simulink model "s_6dof2016a"  (R2016a)
settings: Solver=VariableStepAuto  SolverMode=SingleTasking  StartTime=0.0  StopTime=90  RelTol=1e-3
(part 2 of 2)

== system s_6dof2016a/Subsystem1/B/b513 ==
  t5 : Inport
  t2 : Inport  Port=2
  t3 : Inport  Port=3
  t4 : Inport  Port=4
  Constant4 : Constant  Value=-1
  Product : Product
  b1 : Subsystem
  b513 : Outport
  wires:
  t5/1 -> b1/3(t5)
  Constant4/1 -> Product/2
  b1/1(b315) -> Product/1
  t4/1 -> b1/2(t4)
  Product/1 -> b513/1
  t2/1 -> b1/1(t2)
  t3/1 -> b1/4(t3)

== system s_6dof2016a/Subsystem1/B/b514 ==
  t2 : Inport
  t3 : Inport  Port=2
  t4 : Inport  Port=3
  Constant3 : Constant  Value=-1
  Product : Product
  b1 : Subsystem
  b514 : Outport
  wires:
  Constant3/1 -> Product/2
  t4/1 -> b1/3(t4)
  t2/1 -> b1/1(t2)
  b1/1(b415) -> Product/1
  Product/1 -> b514/1
  t3/1 -> b1/2(t3)

== system s_6dof2016a/Subsystem1/B/b523 ==
  t5 : Inport
  Constant3 : Constant  Value=-1
  Product1 : Product
  b1 : Subsystem
  b523 : Outport
  wires:
  b1/1(b325) -> Product1/1
  t5/1 -> b1/1(t5)
  Constant3/1 -> Product1/2
  Product1/1 -> b523/1

== system s_6dof2016a/Subsystem1/B/b524 ==
  t4 : Inport
  Constant3 : Constant  Value=-1
  Product1 : Product
  b1 : Subsystem
  b524 : Outport
  wires:
  b1/1(b425) -> Product1/1
  t4/1 -> b1/1(t4)
  Product1/1 -> b524/1
  Constant3/1 -> Product1/2

== system s_6dof2016a/Subsystem1/B/b534 ==
  t4 : Inport
  Constant3 : Constant  Value=-1
  Product1 : Product
  b1 : Subsystem
  b524 : Outport
  wires:
  Constant3/1 -> Product1/2
  Product1/1 -> b524/1
  t4/1 -> b1/1(t4)
  b1/1(b425) -> Product1/1

== system s_6dof2016a/Subsystem1/C/c12 ==
  t2 : Inport
  t3 : Inport  Port=2
  Add1 : Sum  Inputs=+++
  Add2 : Sum
  Product1 : Product
  Product3 : Product
  Product4 : Product
  Trigonometric Function1 : Trigonometry  Operator=cos
  Trigonometric Function4 : Trigonometry
  Trigonometric Function5 : Trigonometry
  c2 : Constant  Value=0.69
  c3 : Constant  Value=0.134
  c4 : Constant  Value=-0.0238
  c12 : Outport
  wires:
  Product1/1 -> Add1/1
  Product4/1 -> Add1/3
  Trigonometric Function1/1 -> Product1/2
  Trigonometric Function4/1 -> Product3/2
  Product3/1 -> Add1/2
  t2/1 -> Trigonometric Function5/1, Add2/1, Trigonometric Function1/1
  Add2/1 -> Trigonometric Function4/1
  Trigonometric Function5/1 -> Product4/2
  t3/1 -> Add2/2
  c2/1 -> Product1/1
  c3/1 -> Product3/1
  c4/1 -> Product4/1
  Add1/1 -> c12/1

== system s_6dof2016a/Subsystem1/C/c13 ==
  t2 : Inport
  "t3 " : Inport  Port=2
  Product1 : Product
  Product2 : Product
  Sum2 : Sum  Inputs=|++
  Sum3 : Sum  Inputs=|++
  Trigonometric Function : Trigonometry
  Trigonometric Function1 : Trigonometry  Operator=cos
  b1 : Constant  Value=0.267
  b2 : Constant  Value=-0.00758
  b123 : Outport
  wires:
  Trigonometric Function/1 -> Product2/2
  Product1/1 -> Sum3/2
  Sum3/1 -> b123/1
  Trigonometric Function1/1 -> Product1/2
  Sum2/1 -> Trigonometric Function1/1, Trigonometric Function/1
  b1/1 -> Product2/1
  Product2/1 -> Sum3/1
  b2/1 -> Product1/1
  "t3 "/1 -> Sum2/2
  t2/1 -> Sum2/1

== system s_6dof2016a/Subsystem1/C/c21 ==
  t2 : Inport
  t3 : Inport  Port=2
  Product1 : Product
  b112 : Subsystem
  c2 : Constant  Value=-0.5
  c21 : Outport
  wires:
  c2/1 -> Product1/2
  Product1/1 -> c21/1
  b112/1(b112) -> Product1/1
  t3/1 -> b112/2(t3)
  t2/1 -> b112/1(t2)

== system s_6dof2016a/Subsystem1/C/c23 ==
  t3 : Inport
  Product2 : Product
  b223 : Subsystem
  c2 : Constant  Value=0.5
  c23 : Outport
  wires:
  b223/1(b223) -> Product2/1
  t3/1 -> b223/1(t3)
  c2/1 -> Product2/2
  Product2/1 -> c23/1

== system s_6dof2016a/Subsystem1/C/c31 ==
  t2 : Inport
  t3 : Inport  Port=2
  Product2 : Product
  b113 : Subsystem
  c2 : Constant  Value=-0.5
  c31 : Outport
  wires:
  b113/1(b113) -> Product2/1
  t2/1 -> b113/1(t2)
  c2/1 -> Product2/2
  Product2/1 -> c31/1
  t3/1 -> b113/2(t3)

== system s_6dof2016a/Subsystem1/C/c32 ==
  t3 : Inport
  Product2 : Product
  c2 : Subsystem
  c3 : Constant  Value=-1
  c32 : Outport
  wires:
  c3/1 -> Product2/2
  c2/1(c23) -> Product2/1
  t3/1 -> c2/1(t3)
  Product2/1 -> c32/1

== system s_6dof2016a/Subsystem1/C/c34 ==
  t4 : Inport
  t5 : Inport  Port=2
  Product2 : Product  Inputs=3
  Trigonometric Function1 : Trigonometry  Operator=cos
  Trigonometric Function4 : Trigonometry
  c2 : Constant  Value=-0.00125
  c34 : Outport
  wires:
  Product2/1 -> c34/1
  Trigonometric Function1/1 -> Product2/2
  c2/1 -> Product2/1
  Trigonometric Function4/1 -> Product2/3
  t4/1 -> Trigonometric Function1/1
  t5/1 -> Trigonometric Function4/1

== system s_6dof2016a/Subsystem1/C/c35 ==
  t4 : Inport
  t5 : Inport  Port=2
  Product2 : Product  Inputs=3
  Trigonometric Function1 : Trigonometry  Operator=cos
  Trigonometric Function4 : Trigonometry
  c2 : Constant  Value=-0.00125
  c34 : Outport
  wires:
  Product2/1 -> c34/1
  Trigonometric Function1/1 -> Product2/2
  c2/1 -> Product2/1
  Trigonometric Function4/1 -> Product2/3
  t4/1 -> Trigonometric Function1/1
  t5/1 -> Trigonometric Function4/1

== system s_6dof2016a/Subsystem1/C/c41 ==
  t2 : Inport
  t3 : Inport  Port=2
  t4 : Inport  Port=3
  t5 : Inport  Port=4
  Product2 : Product
  b114 : Subsystem
  c2 : Constant  Value=-0.5
  c41 : Outport
  wires:
  c2/1 -> Product2/2
  t2/1 -> b114/3(t2)
  b114/1(b114) -> Product2/1
  t4/1 -> b114/1(t4)
  Product2/1 -> c41/1
  t3/1 -> b114/4(t3)
  t5/1 -> b114/2(t5)

== system s_6dof2016a/Subsystem1/C/c42 ==
  t3 : Inport
  t4 : Inport  Port=2
  t5 : Inport  Port=3
  Product2 : Product
  b224 : Subsystem
  c2 : Constant  Value=-0.5
  c42 : Outport
  wires:
  t3/1 -> b224/3(t3)
  c2/1 -> Product2/2
  b224/1(b224) -> Product2/1
  t4/1 -> b224/1(t4)
  t5/1 -> b224/2(t5)
  Product2/1 -> c42/1

== system s_6dof2016a/Subsystem1/C/c51 ==
  t2 : Inport
  t3 : Inport  Port=2
  t4 : Inport  Port=3
  t5 : Inport  Port=4
  Product2 : Product
  b115 : Subsystem
  c2 : Constant  Value=-0.5
  c51 : Outport
  wires:
  t5/1 -> b115/2(t5)
  c2/1 -> Product2/2
  b115/1(b115) -> Product2/1
  Product2/1 -> c51/1
  t3/1 -> b115/4(t3)
  t2/1 -> b115/3(t2)
  t4/1 -> b115/1(t4)

== system s_6dof2016a/Subsystem1/C/c52 ==
  t3 : Inport
  t4 : Inport  Port=2
  t5 : Inport  Port=3
  Product2 : Product
  b225 : Subsystem
  c2 : Constant  Value=-0.5
  c52 : Outport
  wires:
  t4/1 -> b225/1(t4)
  b225/1(b225) -> Product2/1
  c2/1 -> Product2/2
  t3/1 -> b225/3(t3)
  Product2/1 -> c52/1
  t5/1 -> b225/2(t5)

== system s_6dof2016a/Subsystem1/C/c53 ==
  t5 : Inport
  Product2 : Product
  b523 : Subsystem
  c2 : Constant  Value=0.5
  c53 : Outport
  wires:
  c2/1 -> Product2/2
  b523/1(b523) -> Product2/1
  t5/1 -> b523/1(t5)
  Product2/1 -> c53/1

== system s_6dof2016a/Subsystem2/Subsystem/a11 ==
  t2 : Inport
  t3 : Inport  Port=2
  Constant3 : Constant  Value=2.57
  Constant4 : Constant  Value=1.38
  Constant5 : Constant  Value=0.3
  Constant6 : Constant  Value=0.744
  Product1 : Product  Inputs=3
  Product2 : Product  Inputs=3
  Product3 : Product  Inputs=3
  Sum : Sum  Inputs=|++
  Sum2 : Sum  Inputs=|++++
  Trigonometric Function1 : Trigonometry  Operator=cos
  Trigonometric Function2 : Trigonometry  Operator=cos
  Trigonometric Function3 : Trigonometry
  Trigonometric Function4 : Trigonometry
  Trigonometric Function5 : Trigonometry
  Trigonometric Function6 : Trigonometry  Operator=cos
  a11 : Outport
  wires:
  Trigonometric Function5/1 -> Product3/1
  Product2/1 -> Sum2/3
  t2/1 -> Trigonometric Function6/1, Sum/1, Trigonometric Function3/1, Trigonometric Function2/1, Trigonometric Function1/1
  t3/1 -> Trigonometric Function4/1, Sum/2
  Constant5/1 -> Product2/3
  Trigonometric Function4/1 -> Product2/2
  Product1/1 -> Sum2/2
  Trigonometric Function3/1 -> Product2/1
  Sum2/1 -> a11/1
  Constant6/1 -> Product3/3
  Trigonometric Function6/1 -> Product3/2
  Sum/1 -> Trigonometric Function5/1
  Constant3/1 -> Sum2/1
  Trigonometric Function1/1 -> Product1/1
  Constant4/1 -> Product1/3
  Trigonometric Function2/1 -> Product1/2
  Product3/1 -> Sum2/4

== system s_6dof2016a/Subsystem2/Subsystem/a12 ==
  t2 : Inport
  t3 : Inport  Port=2
  Constant3 : Constant  Value=0.69
  Constant4 : Constant  Value=0.134
  Constant5 : Constant  Value=0.0238
  Product1 : Product
  Product2 : Product
  Product3 : Product
  Sum1 : Sum  Inputs=|++
  Sum3 : Sum  Inputs=|+-+
  Trigonometric Function1 : Trigonometry
  Trigonometric Function2 : Trigonometry  Operator=cos
  Trigonometric Function3 : Trigonometry  Operator=cos
  a12 : Outport
  wires:
  Constant4/1 -> Product2/1
  t2/1 -> Trigonometric Function3/1, Sum1/1, Trigonometric Function1/1
  Trigonometric Function1/1 -> Product1/2
  Product2/1 -> Sum3/2
  Constant5/1 -> Product3/1
  Product1/1 -> Sum3/1
  Product3/1 -> Sum3/3
  Constant3/1 -> Product1/1
  Sum3/1 -> a12/1
  Trigonometric Function3/1 -> Product3/2
  Sum1/1 -> Trigonometric Function2/1
  Trigonometric Function2/1 -> Product2/2
  t3/1 -> Sum1/2

== system s_6dof2016a/Subsystem2/Subsystem/a13 ==
  "t2 " : Inport
  "t3 " : Inport  Port=2
  Constant3 : Constant  Value=0.134
  Constant4 : Constant  Value=0.00397
  Product : Product
  Product1 : Product
  Sum1 : Sum  Inputs=|++
  Sum3 : Sum  Inputs=|--
  Trigonometric Function1 : Trigonometry  Operator=cos
  Trigonometric Function2 : Trigonometry
  "a13 " : Outport
  wires:
  Product/1 -> Sum3/1
  Sum1/1 -> Trigonometric Function2/1, Trigonometric Function1/1
  Product1/1 -> Sum3/2
  Constant4/1 -> Product1/1
  Constant3/1 -> Product/1
  "t2 "/1 -> Sum1/2
  Trigonometric Function2/1 -> Product1/2
  Trigonometric Function1/1 -> Product/2
  Sum3/1 -> "a13 "/1
  "t3 "/1 -> Sum1/1

== system s_6dof2016a/Subsystem2/Subsystem/a21 ==
  t2 : Inport
  t3 : Inport  Port=2
  Constant3 : Constant  Value=0.69
  Constant4 : Constant  Value=0.134
  Constant5 : Constant  Value=0.0238
  Product1 : Product
  Product2 : Product
  Product3 : Product
  Sum1 : Sum  Inputs=|++
  Sum3 : Sum  Inputs=|+-+
  Trigonometric Function1 : Trigonometry
  Trigonometric Function2 : Trigonometry  Operator=cos
  Trigonometric Function3 : Trigonometry  Operator=cos
  a12 : Outport
  wires:
  Constant4/1 -> Product2/1
  t2/1 -> Trigonometric Function3/1, Sum1/1, Trigonometric Function1/1
  Trigonometric Function1/1 -> Product1/2
  Product2/1 -> Sum3/2
  Constant5/1 -> Product3/1
  Product1/1 -> Sum3/1
  Product3/1 -> Sum3/3
  Constant3/1 -> Product1/1
  Sum3/1 -> a12/1
  Trigonometric Function3/1 -> Product3/2
  Sum1/1 -> Trigonometric Function2/1
  Trigonometric Function2/1 -> Product2/2
  t3/1 -> Sum1/2

== system s_6dof2016a/Subsystem2/Subsystem/a22 ==
  t3 : Inport
  Constant3 : Constant  Value=6.79
  Constant4 : Constant  Value=0.744
  Product1 : Product
  Sum1 : Sum  Inputs=|++
  Trigonometric Function1 : Trigonometry
  a22 : Outport
  wires:
  t3/1 -> Trigonometric Function1/1
  Trigonometric Function1/1 -> Product1/1
  Constant4/1 -> Product1/2
  Product1/1 -> Sum1/1
  Sum1/1 -> a22/1
  Constant3/1 -> Sum1/2

== system s_6dof2016a/Subsystem2/Subsystem/a23 ==
  "t3 " : Inport
  Constant3 : Constant  Value=0.333
  Constant4 : Constant  Value=0.372
  Constant5 : Constant  Value=0.011
  Product1 : Product
  Product2 : Product
  Sum1 : Sum  Inputs=|++-
  Trigonometric Function2 : Trigonometry
  Trigonometric Function3 : Trigonometry  Operator=cos
  a23 : Outport
  wires:
  Constant5/1 -> Product1/1
  Trigonometric Function3/1 -> Product1/2
  Product2/1 -> Sum1/2
  Constant3/1 -> Sum1/1
  "t3 "/1 -> Trigonometric Function3/1, Trigonometric Function2/1
  Product1/1 -> Sum1/3
  Trigonometric Function2/1 -> Product2/2
  Constant4/1 -> Product2/1
  Sum1/1 -> a23/1

== system s_6dof2016a/Subsystem2/Subsystem/a31 ==
  "t2 " : Inport
  "t3 " : Inport  Port=2
  Constant3 : Constant  Value=0.134
  Constant4 : Constant  Value=0.00397
  Product : Product
  Product1 : Product
  Sum1 : Sum  Inputs=|++
  Sum3 : Sum  Inputs=|--
  Trigonometric Function1 : Trigonometry  Operator=cos
  Trigonometric Function2 : Trigonometry
  "a13 " : Outport
  wires:
  Product/1 -> Sum3/1
  Sum1/1 -> Trigonometric Function2/1, Trigonometric Function1/1
  Product1/1 -> Sum3/2
  Constant4/1 -> Product1/1
  Constant3/1 -> Product/1
  "t2 "/1 -> Sum1/2
  Trigonometric Function2/1 -> Product1/2
  Trigonometric Function1/1 -> Product/2
  Sum3/1 -> "a13 "/1
  "t3 "/1 -> Sum1/1

== system s_6dof2016a/Subsystem2/Subsystem/a32 ==
  "t3 " : Inport
  Constant3 : Constant  Value=0.333
  Constant4 : Constant  Value=0.372
  Constant5 : Constant  Value=0.011
  Product1 : Product
  Product2 : Product
  Sum1 : Sum  Inputs=|++-
  Trigonometric Function2 : Trigonometry
  Trigonometric Function3 : Trigonometry  Operator=cos
  a23 : Outport
  wires:
  Constant5/1 -> Product1/1
  Trigonometric Function3/1 -> Product1/2
  Product2/1 -> Sum1/2
  Constant3/1 -> Sum1/1
  "t3 "/1 -> Trigonometric Function3/1, Trigonometric Function2/1
  Product1/1 -> Sum1/3
  Trigonometric Function2/1 -> Product2/2
  Constant4/1 -> Product2/1
  Sum1/1 -> a23/1

== system s_6dof2016a/Subsystem2/Subsystem/a34 ==
  t4 : Inport
  t5 : Inport  Port=2
  Product1 : Product  Inputs=3
  Trigonometric Function1 : Trigonometry
  Trigonometric Function2 : Trigonometry
  a1 : Constant  Value=-0.00125
  a34 : Outport
  wires:
  Trigonometric Function2/1 -> Product1/3
  t4/1 -> Trigonometric Function1/1
  Trigonometric Function1/1 -> Product1/2
  Product1/1 -> a34/1
  a1/1 -> Product1/1
  t5/1 -> Trigonometric Function2/1

== system s_6dof2016a/Subsystem2/Subsystem/a35 ==
  t5 : Inport
  "t4 " : Inport  Port=2
  Product1 : Product  Inputs=3
  Trigonometric Function1 : Trigonometry  Operator=cos
  Trigonometric Function2 : Trigonometry  Operator=cos
  a1 : Constant  Value=0.00125
  a35 : Outport
  wires:
  a1/1 -> Product1/1
  Trigonometric Function1/1 -> Product1/2
  Trigonometric Function2/1 -> Product1/3
  "t4 "/1 -> Trigonometric Function1/1
  Product1/1 -> a35/1
  t5/1 -> Trigonometric Function2/1

== system s_6dof2016a/Subsystem2/Subsystem/a43 ==
  t4 : Inport
  t5 : Inport  Port=2
  Product1 : Product  Inputs=3
  Trigonometric Function1 : Trigonometry
  Trigonometric Function2 : Trigonometry
  a1 : Constant  Value=-0.00125
  a34 : Outport
  wires:
  t5/1 -> Trigonometric Function2/1
  a1/1 -> Product1/1
  Product1/1 -> a34/1
  Trigonometric Function1/1 -> Product1/2
  t4/1 -> Trigonometric Function1/1
  Trigonometric Function2/1 -> Product1/3

== system s_6dof2016a/Subsystem2/Subsystem/a53 ==
  t5 : Inport
  "t4 " : Inport  Port=2
  Product1 : Product  Inputs=3
  Trigonometric Function1 : Trigonometry  Operator=cos
  Trigonometric Function2 : Trigonometry  Operator=cos
  a1 : Constant  Value=0.00125
  a35 : Outport
  wires:
  a1/1 -> Product1/1
  Trigonometric Function1/1 -> Product1/2
  Trigonometric Function2/1 -> Product1/3
  "t4 "/1 -> Trigonometric Function1/1
  Product1/1 -> a35/1
  t5/1 -> Trigonometric Function2/1

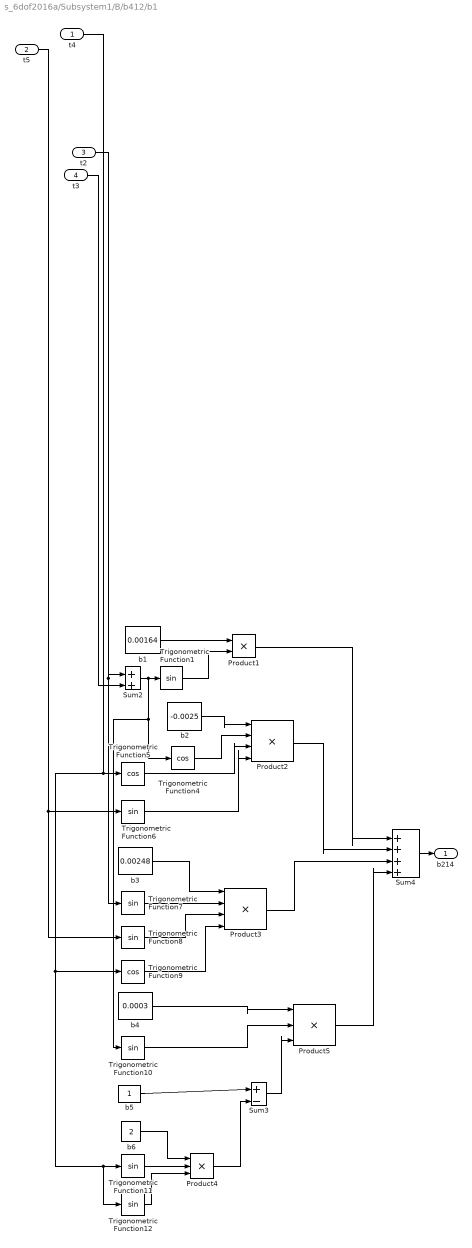
== system s_6dof2016a/Subsystem1/B/b412/b1 ==
  t4 : Inport
  t5 : Inport  Port=2
  t2 : Inport  Port=3
  t3 : Inport  Port=4
  Product1 : Product
  Product2 : Product  Inputs=4
  Product3 : Product  Inputs=4
  Product4 : Product  Inputs=3
  Product5 : Product  Inputs=3
  Sum2 : Sum  Inputs=|++
  Sum3 : Sum  Inputs=|+-
  Sum4 : Sum  Inputs=|++++
  Trigonometric Function{1,6..8,10..12} (7 alike) : Trigonometry
  Trigonometric Function4 : Trigonometry  Operator=cos
  Trigonometric Function5 : Trigonometry  Operator=cos
  Trigonometric Function9 : Trigonometry  Operator=cos
  b1 : Constant  Value=0.00164
  b2 : Constant  Value=-0.0025
  b3 : Constant  Value=0.00248
  b4 : Constant  Value=0.0003
  b5 : Constant
  b6 : Constant  Value=2
  b214 : Outport
  wires:
  Sum2/1 -> Trigonometric Function10/1, Trigonometric Function4/1, Trigonometric Function1/1
  Trigonometric Function5/1 -> Product2/3
  Trigonometric Function1/1 -> Product1/2
  Trigonometric Function6/1 -> Product2/4
  Trigonometric Function10/1 -> Product5/2
  t2/1 -> Trigonometric Function7/1, Sum2/1
  t5/1 -> Trigonometric Function8/1, Trigonometric Function6/1
  b1/1 -> Product1/1
  Trigonometric Function4/1 -> Product2/2
  b6/1 -> Product4/1
  t4/1 -> Trigonometric Function12/1, Trigonometric Function11/1, Trigonometric Function9/1, Trigonometric Function5/1
  Product2/1 -> Sum4/2
  b2/1 -> Product2/1
  b5/1 -> Sum3/1
  Trigonometric Function11/1 -> Product4/2
  Trigonometric Function9/1 -> Product3/4
  Sum3/1 -> Product5/3
  b3/1 -> Product3/1
  Trigonometric Function7/1 -> Product3/2
  Trigonometric Function12/1 -> Product4/3
  b4/1 -> Product5/1
  Trigonometric Function8/1 -> Product3/3
  Product1/1 -> Sum4/1
  Product3/1 -> Sum4/3
  Product4/1 -> Sum3/2
  Sum4/1 -> b214/1
  Product5/1 -> Sum4/4
  t3/1 -> Sum2/2

== system s_6dof2016a/Subsystem1/B/b413/b1 ==
  t2 : Inport
  t4 : Inport  Port=2
  t5 : Inport  Port=3
  t3 : Inport  Port=4
  Constant3 : Constant  Value=0.00164
  Constant4 : Constant  Value=0.0003
  Constant5 : Constant  Value=2
  Constant6 : Constant
  Product1 : Product  Inputs=4
  Product2 : Product
  Product3 : Product  Inputs=3
  Product4 : Product  Inputs=3
  Sum2 : Sum  Inputs=|++
  Sum3 : Sum  Inputs=|+-
  Sum4 : Sum  Inputs=|+++
  Trigonometric Function1 : Trigonometry  Operator=cos
  Trigonometric Function4 : Trigonometry  Operator=cos
  Trigonometric Function{5..9} (5 alike) : Trigonometry
  b1 : Constant  Value=-0.0025
  b314 : Outport
  wires:
  t5/1 -> Trigonometric Function5/1
  Sum4/1 -> b314/1
  Sum2/1 -> Trigonometric Function7/1, Trigonometric Function6/1, Trigonometric Function1/1
  Product1/1 -> Sum4/1
  Constant5/1 -> Product3/1
  b1/1 -> Product1/1
  Product2/1 -> Sum4/2
  Trigonometric Function7/1 -> Product4/2
  Trigonometric Function9/1 -> Product3/3
  t4/1 -> Trigonometric Function4/1, Trigonometric Function9/1, Trigonometric Function8/1
  Sum3/1 -> Product4/3
  Trigonometric Function5/1 -> Product1/4
  Constant3/1 -> Product2/1
  Trigonometric Function6/1 -> Product2/2
  Trigonometric Function1/1 -> Product1/2
  Trigonometric Function4/1 -> Product1/3
  Product3/1 -> Sum3/2
  Product4/1 -> Sum4/3
  Constant6/1 -> Sum3/1
  Trigonometric Function8/1 -> Product3/2
  Constant4/1 -> Product4/1
  t3/1 -> Sum2/2
  t2/1 -> Sum2/1

== system s_6dof2016a/Subsystem1/B/b512/b1 ==
  t4 : Inport
  t5 : Inport  Port=2
  t2 : Inport  Port=3
  t3 : Inport  Port=4
  Product1 : Product  Inputs=4
  Product2 : Product  Inputs=4
  Product3 : Product  Inputs=3
  Sum2 : Sum  Inputs=|++
  Sum3 : Sum  Inputs=|+++
  Trigonometric Function{1,4,8..9} (4 alike) : Trigonometry  Operator=cos
  Trigonometric Function{5..7,10} (4 alike) : Trigonometry
  b1 : Constant  Value=-0.0025
  b2 : Constant  Value=0.00248
  b3 : Constant  Value=-0.000642
  b215 : Outport
  wires:
  t4/1 -> Trigonometric Function10/1, Trigonometric Function7/1, Trigonometric Function5/1
  Trigonometric Function7/1 -> Product2/3
  Trigonometric Function1/1 -> Product1/2
  Trigonometric Function4/1 -> Product1/4
  Trigonometric Function8/1 -> Product2/4
  Trigonometric Function6/1 -> Product2/2
  b2/1 -> Product2/1
  t5/1 -> Trigonometric Function8/1, Trigonometric Function4/1
  t2/1 -> Trigonometric Function6/1, Sum2/1
  Trigonometric Function5/1 -> Product1/3
  Product2/1 -> Sum3/2
  Sum2/1 -> Trigonometric Function9/1, Trigonometric Function1/1
  Product3/1 -> Sum3/3
  Product1/1 -> Sum3/1
  Trigonometric Function9/1 -> Product3/2
  b3/1 -> Product3/1
  Trigonometric Function10/1 -> Product3/3
  b1/1 -> Product1/1
  t3/1 -> Sum2/2
  Sum3/1 -> b215/1

== system s_6dof2016a/Subsystem1/B/b513/b1 ==
  t2 : Inport
  t4 : Inport  Port=2
  t5 : Inport  Port=3
  t3 : Inport  Port=4
  Product1 : Product  Inputs=4
  Product2 : Product  Inputs=3
  Sum2 : Sum  Inputs=|++
  Sum3 : Sum  Inputs=|++
  Trigonometric Function1 : Trigonometry  Operator=cos
  Trigonometric Function4 : Trigonometry  Operator=cos
  Trigonometric Function5 : Trigonometry
  Trigonometric Function6 : Trigonometry  Operator=cos
  Trigonometric Function7 : Trigonometry
  b1 : Constant  Value=-0.0025
  b2 : Constant  Value=-0.000642
  b315 : Outport
  wires:
  Sum2/1 -> Trigonometric Function6/1, Trigonometric Function1/1
  Trigonometric Function4/1 -> Product1/4
  Trigonometric Function5/1 -> Product1/3
  Product1/1 -> Sum3/1
  Trigonometric Function1/1 -> Product1/2
  Product2/1 -> Sum3/2
  t3/1 -> Sum2/2
  Sum3/1 -> b315/1
  t4/1 -> Trigonometric Function7/1, Trigonometric Function5/1
  t2/1 -> Sum2/1
  Trigonometric Function7/1 -> Product2/3
  b2/1 -> Product2/1
  Trigonometric Function6/1 -> Product2/2
  b1/1 -> Product1/1
  t5/1 -> Trigonometric Function4/1

== system s_6dof2016a/Subsystem1/B/b514/b1 ==
  t2 : Inport
  t3 : Inport  Port=2
  t4 : Inport  Port=3
  Constant3 : Constant  Value=-0.000642
  Product1 : Product  Inputs=3
  Sum2 : Sum  Inputs=|++
  Trigonometric Function1 : Trigonometry  Operator=cos
  Trigonometric Function4 : Trigonometry
  b415 : Outport
  wires:
  Trigonometric Function4/1 -> Product1/2
  t4/1 -> Trigonometric Function1/1
  Trigonometric Function1/1 -> Product1/3
  t3/1 -> Sum2/2
  Product1/1 -> b415/1
  t2/1 -> Sum2/1
  Constant3/1 -> Product1/1
  Sum2/1 -> Trigonometric Function4/1

== system s_6dof2016a/Subsystem1/B/b523/b1 ==
  t5 : Inport
  Product1 : Product
  Trigonometric Function1 : Trigonometry
  b1 : Constant  Value=-0.0025
  b325 : Outport
  wires:
  Trigonometric Function1/1 -> Product1/2
  b1/1 -> Product1/1
  Product1/1 -> b325/1
  t5/1 -> Trigonometric Function1/1

== system s_6dof2016a/Subsystem1/B/b524/b1 ==
  t4 : Inport
  Product1 : Product
  Trigonometric Function1 : Trigonometry
  b1 : Constant  Value=0.000642
  b425 : Outport
  wires:
  Trigonometric Function1/1 -> Product1/2
  b1/1 -> Product1/1
  t4/1 -> Trigonometric Function1/1
  Product1/1 -> b425/1

== system s_6dof2016a/Subsystem1/B/b534/b1 ==
  t4 : Inport
  Product1 : Product
  Trigonometric Function1 : Trigonometry
  b1 : Constant  Value=0.000642
  b425 : Outport
  wires:
  Product1/1 -> b425/1
  t4/1 -> Trigonometric Function1/1
  b1/1 -> Product1/1
  Trigonometric Function1/1 -> Product1/2

== system s_6dof2016a/Subsystem1/C/c21/b112 ==
  t2 : Inport
  t3 : Inport  Port=2
  Constant3 : Constant  Value=-2.76
  Constant4 : Constant  Value=0.6
  Constant5 : Constant  Value=0.744
  Constant6 : Constant  Value=-0.0213
  Constant7 : Constant
  Constant8 : Constant  Value=2
  Product1 : Product  Inputs=3
  Product2 : Product  Inputs=3
  Product3 : Product  Inputs=3
  Product4 : Product
  Product5 : Product
  Sum1 : Sum  Inputs=|++
  Sum3 : Sum  Inputs=|+++
  Sum4 : Sum  Inputs=|+-
  Sum5 : Sum  Inputs=|++++
  Trigonometric Function{1,4,6,8} (4 alike) : Trigonometry
  Trigonometric Function2 : Trigonometry  Operator=cos
  Trigonometric Function5 : Trigonometry  Operator=cos
  Trigonometric Function7 : Trigonometry  Operator=cos
  b112 : Outport
  wires:
  t2/1 -> Sum3/1, Sum1/1, Trigonometric Function1/1, Trigonometric Function2/1
  Trigonometric Function1/1 -> Product1/2
  Trigonometric Function8/1 -> Product3/3
  t3/1 -> Sum3/3, Sum3/2, Sum1/2
  Constant5/1 -> Product5/2
  Sum5/1 -> b112/1
  Product3/1 -> Sum4/2
  Constant3/1 -> Product1/1
  Sum1/1 -> Trigonometric Function8/1, Trigonometric Function6/1, Trigonometric Function5/1, Trigonometric Function4/1
  Constant6/1 -> Product4/1
  Constant8/1 -> Product3/1
  Trigonometric Function7/1 -> Product5/1
  Constant4/1 -> Product2/1
  Constant7/1 -> Sum4/1
  Trigonometric Function5/1 -> Product2/3
  Product4/1 -> Sum5/4
  Product2/1 -> Sum5/2
  Trigonometric Function2/1 -> Product1/3
  Trigonometric Function6/1 -> Product3/2
  Trigonometric Function4/1 -> Product2/2
  Sum3/1 -> Trigonometric Function7/1
  Product1/1 -> Sum5/1
  Sum4/1 -> Product4/2
  Product5/1 -> Sum5/3

== system s_6dof2016a/Subsystem1/C/c23/b223 ==
  t3 : Inport
  Product1 : Product
  Product2 : Product
  Sum2 : Sum  Inputs=|++
  Trigonometric Function1 : Trigonometry
  Trigonometric Function4 : Trigonometry  Operator=cos
  b1 : Constant  Value=0.022
  b2 : Constant  Value=0.744
  b223 : Outport
  wires:
  Sum2/1 -> b223/1
  b1/1 -> Product1/1
  b2/1 -> Product2/1
  Product2/1 -> Sum2/2
  t3/1 -> Trigonometric Function4/1, Trigonometric Function1/1
  Product1/1 -> Sum2/1
  Trigonometric Function4/1 -> Product2/2
  Trigonometric Function1/1 -> Product1/2

== system s_6dof2016a/Subsystem1/C/c31/b113 ==
  t2 : Inport
  t3 : Inport  Port=2
  Constant3 : Constant  Value=0.744
  Constant4 : Constant  Value=0.6
  Constant5 : Constant  Value=0.022
  Constant6 : Constant  Value=-0.0213
  Constant7 : Constant
  Constant8 : Constant  Value=2
  Product{1..4} (4 alike) : Product  Inputs=3
  Product5 : Product
  Sum1 : Sum  Inputs=|++
  Sum3 : Sum  Inputs=|++++
  Sum4 : Sum  Inputs=|+-
  Trigonometric Function{1..2,5..6} (4 alike) : Trigonometry  Operator=cos
  Trigonometric Function{4,7..9} (4 alike) : Trigonometry
  b113 : Outport
  wires:
  Product2/1 -> Sum3/2
  t2/1 -> Trigonometric Function6/1, Sum1/1, Trigonometric Function1/1
  Trigonometric Function5/1 -> Product2/3
  Trigonometric Function1/1 -> Product1/2
  Constant3/1 -> Product1/1
  t3/1 -> Sum1/2
  Constant4/1 -> Product2/1
  Sum1/1 -> Trigonometric Function9/1, Trigonometric Function8/1, Trigonometric Function7/1, Trigonometric Function5/1, Trigonometric Function4/1, Trigonometric Function2/1
  Product3/1 -> Sum3/3
  Trigonometric Function9/1 -> Product4/3
  Constant6/1 -> Product5/1
  Trigonometric Function2/1 -> Product1/3
  Sum4/1 -> Product5/2
  Trigonometric Function8/1 -> Product4/2
  Sum3/1 -> b113/1
  Trigonometric Function7/1 -> Product3/2
  Constant8/1 -> Product4/1
  Constant7/1 -> Sum4/1
  Product4/1 -> Sum4/2
  Product5/1 -> Sum3/4
  Product1/1 -> Sum3/1
  Trigonometric Function4/1 -> Product2/2
  Trigonometric Function6/1 -> Product3/3
  Constant5/1 -> Product3/1

== system s_6dof2016a/Subsystem1/C/c32/c2 ==
  t3 : Inport
  Product2 : Product
  b223 : Subsystem
  c2 : Constant  Value=0.5
  c23 : Outport
  wires:
  b223/1(b223) -> Product2/1
  t3/1 -> b223/1(t3)
  c2/1 -> Product2/2
  Product2/1 -> c23/1

== system s_6dof2016a/Subsystem1/C/c41/b114 ==
  t4 : Inport
  t5 : Inport  Port=2
  t2 : Inport  Port=3
  t3 : Inport  Port=4
  Constant3 : Constant  Value=-0.0025
  Constant4 : Constant  Value=0.00086
  Constant5 : Constant  Value=-0.00248
  Product1 : Product  Inputs=5
  Product2 : Product  Inputs=3
  Product3 : Product  Inputs=5
  Sum1 : Sum  Inputs=|++
  Sum3 : Sum  Inputs=|+++
  Trigonometric Function{1..2,4,7,10..11} (6 alike) : Trigonometry
  Trigonometric Function{5..6,8..9} (4 alike) : Trigonometry  Operator=cos
  b114 : Outport
  wires:
  t2/1 -> Sum1/1, Trigonometric Function9/1
  Trigonometric Function1/1 -> Product1/2
  t4/1 -> Trigonometric Function11/1, Trigonometric Function6/1, Trigonometric Function2/1
  Product1/1 -> Sum3/1
  Trigonometric Function11/1 -> Product3/4
  Trigonometric Function4/1 -> Product1/5
  Constant3/1 -> Product1/1
  t5/1 -> Trigonometric Function10/1, Trigonometric Function7/1, Trigonometric Function4/1
  Trigonometric Function10/1 -> Product3/5
  Trigonometric Function5/1 -> Product1/3
  Sum1/1 -> Trigonometric Function8/1, Trigonometric Function5/1, Trigonometric Function1/1
  Trigonometric Function8/1 -> Product3/2
  Trigonometric Function2/1 -> Product1/4
  Trigonometric Function9/1 -> Product3/3
  Constant5/1 -> Product3/1
  Trigonometric Function7/1 -> Product2/3
  Product3/1 -> Sum3/3
  Product2/1 -> Sum3/2
  Constant4/1 -> Product2/1
  Trigonometric Function6/1 -> Product2/2
  t3/1 -> Sum1/2
  Sum3/1 -> b114/1

== system s_6dof2016a/Subsystem1/C/c42/b224 ==
  t4 : Inport
  t5 : Inport  Port=2
  t3 : Inport  Port=3
  Product1 : Product  Inputs=4
  Trigonometric Function1 : Trigonometry  Operator=cos
  Trigonometric Function4 : Trigonometry
  Trigonometric Function5 : Trigonometry
  b1 : Constant  Value=-0.00248
  b224 : Outport
  wires:
  Trigonometric Function1/1 -> Product1/2
  Trigonometric Function5/1 -> Product1/4
  t5/1 -> Trigonometric Function5/1
  Trigonometric Function4/1 -> Product1/3
  b1/1 -> Product1/1
  Product1/1 -> b224/1
  t4/1 -> Trigonometric Function4/1
  t3/1 -> Trigonometric Function1/1

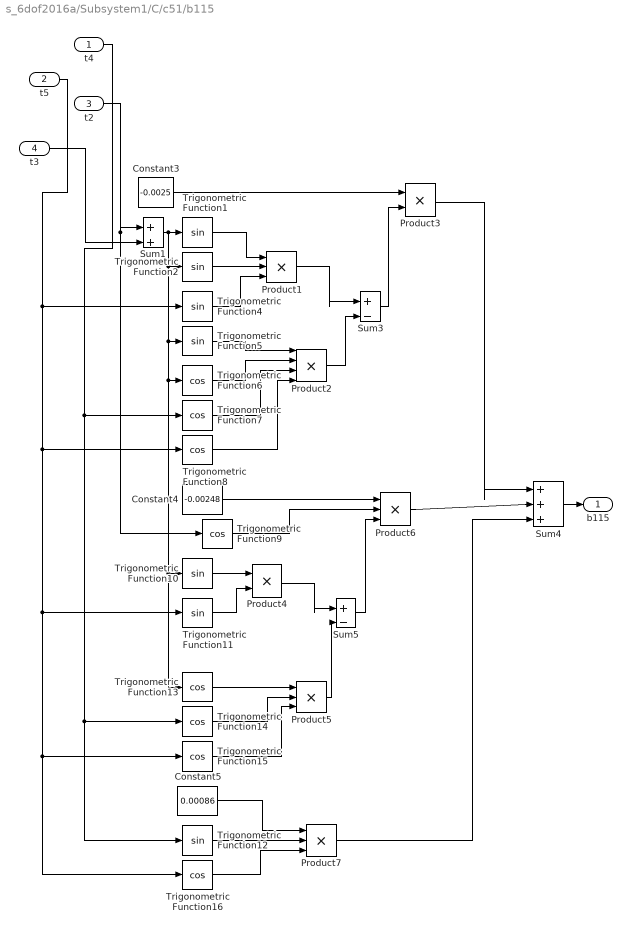
== system s_6dof2016a/Subsystem1/C/c51/b115 ==
  t4 : Inport
  t5 : Inport  Port=2
  t2 : Inport  Port=3
  t3 : Inport  Port=4
  Constant3 : Constant  Value=-0.0025
  Constant4 : Constant  Value=-0.00248
  Constant5 : Constant  Value=0.00086
  Product{1,5..7} (4 alike) : Product  Inputs=3
  Product2 : Product  Inputs=4
  Product3 : Product
  Product4 : Product
  Sum1 : Sum  Inputs=|++
  Sum3 : Sum  Inputs=|+-
  Sum4 : Sum  Inputs=|+++
  Sum5 : Sum  Inputs=|+-
  Trigonometric Function{1..2,4..5,10..12} (7 alike) : Trigonometry
  Trigonometric Function{6..9,13..16} (8 alike) : Trigonometry  Operator=cos
  b115 : Outport
  wires:
  Trigonometric Function2/1 -> Product1/2
  Sum1/1 -> Trigonometric Function13/1, Trigonometric Function10/1, Trigonometric Function6/1, Trigonometric Function5/1, Trigonometric Function2/1, Trigonometric Function1/1
  Sum3/1 -> Product3/2
  Trigonometric Function16/1 -> Product7/3
  Trigonometric Function5/1 -> Product2/1
  Trigonometric Function4/1 -> Product1/3
  t4/1 -> Trigonometric Function12/1, Trigonometric Function14/1, Trigonometric Function7/1
  Product1/1 -> Sum3/1
  Product2/1 -> Sum3/2
  t5/1 -> Trigonometric Function16/1, Trigonometric Function15/1, Trigonometric Function11/1, Trigonometric Function8/1, Trigonometric Function4/1
  Trigonometric Function12/1 -> Product7/2
  Trigonometric Function6/1 -> Product2/2
  Trigonometric Function14/1 -> Product5/2
  t3/1 -> Sum1/2
  Product3/1 -> Sum4/1
  Product4/1 -> Sum5/1
  Trigonometric Function15/1 -> Product5/3
  Trigonometric Function10/1 -> Product4/1
  Trigonometric Function8/1 -> Product2/4
  Product6/1 -> Sum4/2
  Product7/1 -> Sum4/3
  Trigonometric Function7/1 -> Product2/3
  t2/1 -> Trigonometric Function9/1, Sum1/1
  Constant5/1 -> Product7/1
  Trigonometric Function1/1 -> Product1/1
  Sum5/1 -> Product6/3
  Trigonometric Function9/1 -> Product6/2
  Constant3/1 -> Product3/1
  Trigonometric Function11/1 -> Product4/2
  Constant4/1 -> Product6/1
  Product5/1 -> Sum5/2
  Trigonometric Function13/1 -> Product5/1
  Sum4/1 -> b115/1

== system s_6dof2016a/Subsystem1/C/c52/b225 ==
  t4 : Inport
  t5 : Inport  Port=2
  t3 : Inport  Port=3
  Constant3 : Constant  Value=-0.0025
  Constant4 : Constant  Value=0.00248
  Product1 : Product
  Product2 : Product  Inputs=3
  Product3 : Product
  Product4 : Product
  Sum2 : Sum  Inputs=|+-
  Sum3 : Sum  Inputs=|++
  Trigonometric Function1 : Trigonometry
  Trigonometric Function4 : Trigonometry  Operator=cos
  Trigonometric Function5 : Trigonometry  Operator=cos
  Trigonometric Function6 : Trigonometry  Operator=cos
  Trigonometric Function7 : Trigonometry
  Trigonometric Function8 : Trigonometry
  b225 : Outport
  wires:
  Sum2/1 -> Product4/2
  t5/1 -> Trigonometric Function8/1, Trigonometric Function6/1, Trigonometric Function1/1
  Trigonometric Function8/1 -> Product3/2
  Constant4/1 -> Product4/1
  Trigonometric Function6/1 -> Product2/3
  Product2/1 -> Sum2/1
  t3/1 -> Trigonometric Function7/1, Trigonometric Function4/1
  Trigonometric Function4/1 -> Product2/1
  Product1/1 -> Sum3/1
  Product4/1 -> Sum3/2
  Constant3/1 -> Product1/1
  Trigonometric Function7/1 -> Product3/1
  Trigonometric Function1/1 -> Product1/2
  Product3/1 -> Sum2/2
  Trigonometric Function5/1 -> Product2/2
  Sum3/1 -> b225/1
  t4/1 -> Trigonometric Function5/1

== system s_6dof2016a/Subsystem1/C/c53/b523 ==
  t5 : Inport
  Constant3 : Constant  Value=-1
  Product1 : Product
  b1 : Subsystem
  b523 : Outport
  wires:
  b1/1(b325) -> Product1/1
  t5/1 -> b1/1(t5)
  Constant3/1 -> Product1/2
  Product1/1 -> b523/1

== system s_6dof2016a/Subsystem1/C/c32/c2/b223 ==
  t3 : Inport
  Product1 : Product
  Product2 : Product
  Sum2 : Sum  Inputs=|++
  Trigonometric Function1 : Trigonometry
  Trigonometric Function4 : Trigonometry  Operator=cos
  b1 : Constant  Value=0.022
  b2 : Constant  Value=0.744
  b223 : Outport
  wires:
  Sum2/1 -> b223/1
  b1/1 -> Product1/1
  b2/1 -> Product2/1
  Product2/1 -> Sum2/2
  t3/1 -> Trigonometric Function4/1, Trigonometric Function1/1
  Product1/1 -> Sum2/1
  Trigonometric Function4/1 -> Product2/2
  Trigonometric Function1/1 -> Product1/2

== system s_6dof2016a/Subsystem1/C/c53/b523/b1 ==
  t5 : Inport
  Product1 : Product
  Trigonometric Function1 : Trigonometry
  b1 : Constant  Value=-0.0025
  b325 : Outport
  wires:
  Trigonometric Function1/1 -> Product1/2
  b1/1 -> Product1/1
  Product1/1 -> b325/1
  t5/1 -> Trigonometric Function1/1
